simulink model "Open_Loop2024"  (R2025b)
settings: Solver=FixedStepAuto  StartTime=0.0  StopTime=10.0  FixedStep=0.0001  RelTol=1e-3  EnableMultiTasking=on
InitFcn:
  | Ts=100e-6;
  | 
  | Pair_poles=5;
  | 
  | PWM_frequesncy=10000;
  | 
  | Base_speed=4000;
  | 
  | motor.base_freq=100;
  | 
  | dataType = Simulink.NumericType;
  | 
  | dataType.DataTypeMode = 'Fixed-point: binary point scaling';
  | 
  | dataType.Signedness = 'Signed';
  | 
  | dataType.WordLength = 32;
  | 
  | dataType.FractionLength = 17;
undefined symbols (not defined in the file): DiscIntNeverNeededParam
libraries: stm32f4xxblockslib x14, stm32blockslib x2, mcbpositiondecoderlib x2, mcbcontrolslib x2, stm32f3xxblockslib x2
settings Model: STM32="{\"HardwareInterrupt\":[{\"ID\":\"Open_Loop2024:7\"},{\"ID\":\"Open_Loop2024:322\"}],\"DigitalPortWrite\":[{\"ID\":\"Open_Loop2024:136\"},{\"ID\":\"Open_Loop2024:394\"},{\"ID\":\"Open_Loop2024:286\"}],\"AnalogInput\":{\"ID\":\"Open_Loop2024:13\"},\"DigitalPortRead\":[{\"ID\":\"Open_Loop2024:219\"},{\"ID\":\"Open_Loop2024:220\"},{\"ID\":\"Open_Loop2024:221\"},{\"ID\":\"Open_Loop2024:342\"},{\"ID\":\"Open_Loop2024:343\"},{\"ID\":\"Open_Loop2024:344\"},{\"ID\":\"Open_Loop2024:366\"},{\"ID\":\"Open_Loop2024:367\"},{\"ID\":\"Open_Loop2024:368\"}],\"PWMOutput\":{\"ID\":\"Open_Loop2024:3\"},\"TimerCapture\":{\"ID\":\"Open_Loop2024:351\"},\"AnalogOutput\":{\"ID\":\"Open_Loop2024:377\"}}"  Creator=be125564  LastModifiedBy=be125564
settings SolverCC: AutoInsertRateTranBlk=on
settings OptimizationCC: DefaultParameterBehavior=Inlined  EnhancedBackFolding=on  PassReuseOutputArgsAs=Individual arguments  ZeroExternalMemoryAtStartup=off  ZeroInternalMemoryAtStartup=off  MaxStackSize=512  OptimizeBlockOrder=speed  DifferentSizesBufferReuse=on  OptimizationCustomize=off  EfficientTunableParamExpr=on
settings DebuggingCC: MultiTaskDSMMsg=warning  ParameterTunabilityLossMsg=error
settings HardwareCC: ProdBitPerPointer=32.0  ProdBitPerSizeT=32.0  ProdBitPerPtrDiffT=32.0  ProdLargestAtomicInteger=Long  ProdLargestAtomicFloat=Double  ProdWordSize=32.0  ProdLongLongMode=on  ProdHWDeviceType=ARM Compatible->ARM Cortex-M
settings SFSimCC: MATLABDynamicMemAlloc=off
settings RTWCC: SystemTargetFile=ert.tlc  HardwareBoard=STM32F3xx Based  TemplateMakefile=ert_default_tmf  Toolchain=GNU Tools for ARM Embedded Processors  Description=Embedded Coder
settings CodeAppCC: ForceParamTrailComments=on  IgnoreCustomStorageClasses=off  OperatorAnnotations=on  SimulinkDataObjDesc=on  SFDataObjDesc=on  InsertBlockDesc=on
settings ERTTargetCC: ExtModeTransport=3.0  ExtModeStaticAlloc=on  ExtModeStaticAllocSize=2048.0  ExtModeMexFile=ext_xcp  ExtModeIntrfLevel=Level2 - Open  DynamicArrayContainerType=coder::array  TargetLangStandard=C99 (ISO)  CodeReplacementLibrary=ARM Cortex-M

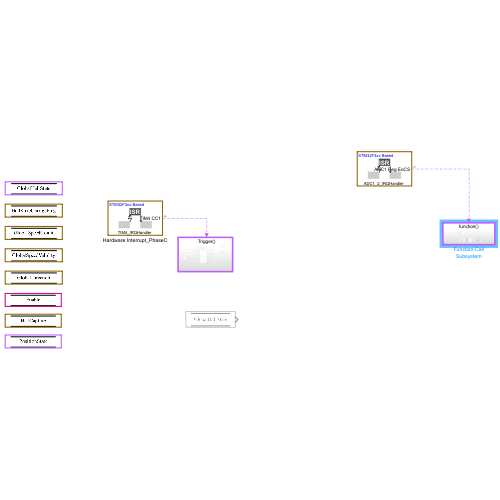
[thumbnail: Simulink's stored preview of the top-level diagram]
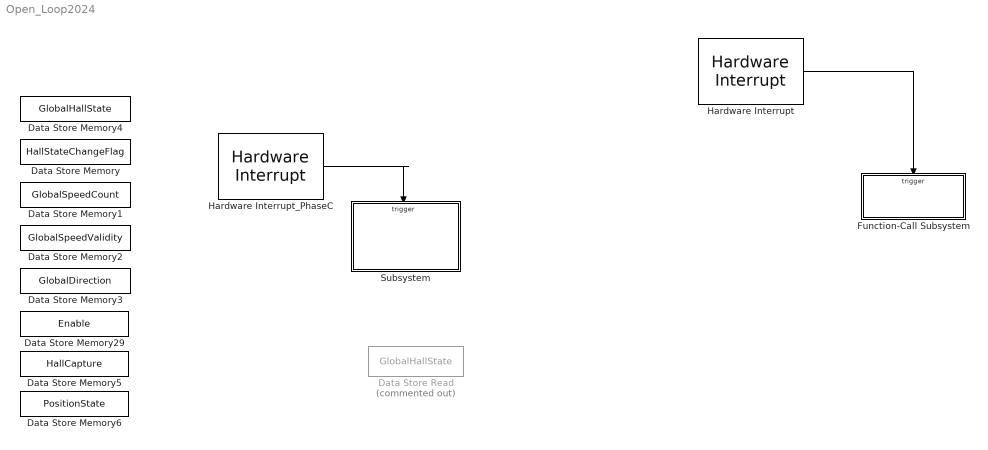
== system Open_Loop2024 ==
  Data Store Memory : DataStoreMemory  DataStoreName=HallStateChangeFlag  ShowAdditionalParam=off
  Data Store Memory1 : DataStoreMemory  DataStoreName=GlobalSpeedCount  ShowAdditionalParam=off
  Data Store Memory2 : DataStoreMemory  DataStoreName=GlobalSpeedValidity  ShowAdditionalParam=off
  Data Store Memory29 : DataStoreMemory  DataStoreName=Enable  ReadBeforeWriteMsg=warning  WriteAfterWriteMsg=warning  WriteAfterReadMsg=warning  ShowAdditionalParam=off  OutDataTypeStr=boolean
  Data Store Memory3 : DataStoreMemory  DataStoreName=GlobalDirection  ShowAdditionalParam=off
  Data Store Memory4 : DataStoreMemory  DataStoreName=GlobalHallState  ShowAdditionalParam=off  OutDataTypeStr=uint32
  Data Store Memory5 : DataStoreMemory  DataStoreName=HallCapture  ReadBeforeWriteMsg=warning  WriteAfterWriteMsg=warning  WriteAfterReadMsg=warning  ShowAdditionalParam=off  OutDataTypeStr=uint16
  Data Store Memory6 : DataStoreMemory  DataStoreName=PositionState  ReadBeforeWriteMsg=warning  WriteAfterWriteMsg=warning  WriteAfterReadMsg=warning  ShowAdditionalParam=off  OutDataTypeStr=uint16
  Data Store Read : DataStoreRead  Commented=on  DataStoreName=GlobalHallState  IndexOptions=Index vector (dialog)  Indices=1  OutputSizes=1
  Function-Call Subsystem : Subsystem  TreatAsAtomicUnit=on
  Hardware Interrupt : stm32f3xxblockslib/Hardware Interrupt  ISRGroup=Analog to digital converter (ADC)  ISRName=ADC1_2_IRQHandler  ISRNumber=33  EventsList={ 'off', 'ADC1 OVR', '1'; 'on', 'ADC1 Reg EoCS', '2'; 'off', 'ADC1 Watchdog1', '3'; 'off', 'ADC1 Watchdog2', '4'; 'off', 'ADC1 Watchdog3', '5'; 'off', 'ADC2 OVR', '6'; 'off', 'ADC2 Reg EoCS', '7'; 'off', 'ADC2 Watchdog1', '8'; 'off', 'ADC2 Watchdog2', '9'; 'off', 'ADC2 Watchdog3', '10'; 'off', 'Custom event', '11' }  SelectedEvents={'ADC1 Reg EoCS'}  TaskPriority=20  DisablePreemption=off  ClearInterruptFlagsAtEndOfEvent=on  InterruptDefinitionFile=$(TARGET_ROOT)/registry/interrupts/STM32F3xxBased_interrupts.xml  HardwareBoard=STM32F3xx Based  EnableSimPort=off
  Hardware Interrupt_PhaseC : stm32f3xxblockslib/Hardware Interrupt  ISRGroup=Timer (TIM)  ISRName=TIM4_IRQHandler  ISRNumber=45  EventsList={ 'off', 'TIM4 Update', '1'; 'on', 'TIM4 CC1', '2'; 'off', 'TIM4 CC2', '3'; 'off', 'TIM4 CC3', '4'; 'off', 'TIM4 CC4', '5'; 'off', 'TIM4 Trigger', '6'; 'off', 'Custom event', '7' }  SelectedEvents={'TIM4 CC1'}  TaskPriority=30  DisablePreemption=off  ClearInterruptFlagsAtEndOfEvent=on  InterruptDefinitionFile=$(TARGET_ROOT)/registry/interrupts/STM32F3xxBased_interrupts.xml  HardwareBoard=STM32F3xx Based  EnableSimPort=off
  Subsystem : Subsystem
  wires:
  Hardware Interrupt/1 -> Function-Call Subsystem/Trigger
  Hardware Interrupt_PhaseC/1 -> Subsystem/Trigger

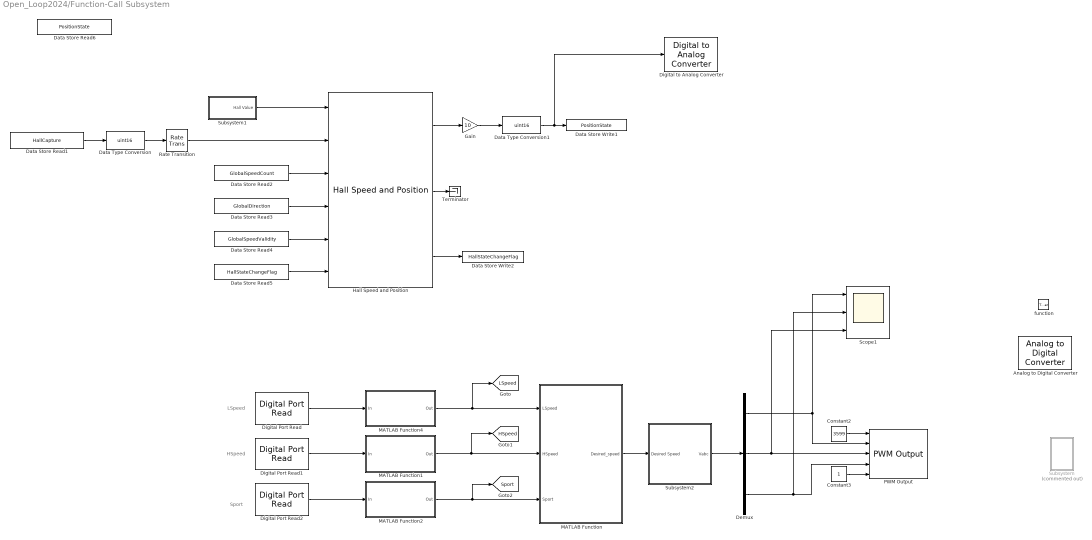
== system Open_Loop2024/Function-Call Subsystem ==
  note: Sport
  note: LSpeed
  note: HSpeed
  function : TriggerPort  TriggerType=function-call  VariantControl=(inherit)
  Analog to Digital Converter : stm32f4xxblockslib/Analog to Digital Converter  ADCModule=ADC1  ConversionGroup=Regular  TriggerMode=Trigger and read  NumberOfConversions=1  EnableBufferConv=off  BufferLength=1  OutputStatus=off  SampleTime=-1  EnableSimPort=off  hoistedMaskSrc=ECSoC/ECSimCodegen/Analog to Digital Converter
      settings: LibrarySourceBlock=stm32f3xxblockslib/Analog to Digital Converter
  Constant2 : Constant  Value=3599  SampleTime=-1
  Constant3 : Constant  SampleTime=-1
  Data Store Read1 : DataStoreRead  DataStoreName=HallCapture  IndexOptions=Index vector (dialog)  Indices=1  OutputSizes=1
  Data Store Read2 : DataStoreRead  DataStoreName=GlobalSpeedCount  IndexOptions=Index vector (dialog)  Indices=1  OutputSizes=1
  Data Store Read3 : DataStoreRead  DataStoreName=GlobalDirection  IndexOptions=Index vector (dialog)  Indices=1  OutputSizes=1
  Data Store Read4 : DataStoreRead  DataStoreName=GlobalSpeedValidity  IndexOptions=Index vector (dialog)  Indices=1  OutputSizes=1
  Data Store Read5 : DataStoreRead  Priority=1  DataStoreName=HallStateChangeFlag  IndexOptions=Index vector (dialog)  Indices=1  OutputSizes=1
  Data Store Read6 : DataStoreRead  DataStoreName=PositionState  IndexOptions=Index vector (dialog)  Indices=1  OutputSizes=1
  Data Store Write1 : DataStoreWrite  DataStoreName=PositionState  IndexOptions=Index vector (dialog)  Indices=1  OutputSizes=1
  Data Store Write2 : DataStoreWrite  DataStoreName=HallStateChangeFlag  IndexOptions=Index vector (dialog)  Indices=1  OutputSizes=1
  Data Type Conversion : DataTypeConversion  OutDataTypeStr=uint16  SaturateOnIntegerOverflow=off  RndMeth=Floor
  Data Type Conversion1 : DataTypeConversion  OutDataTypeStr=uint16  SaturateOnIntegerOverflow=off  RndMeth=Floor
  Demux : Demux  Outputs=3
  Digital Port Read : stm32f4xxblockslib/Digital Port Read  PortName=GPIOC  PinNumber=[6]  ReadOperation=on  IOAsArray=on  SampleTime=-1  EnableSimPort=off  hoistedMaskSrc=ECSoC/ECSimCodegen/Digital Port Read
  Digital Port Read1 : stm32f4xxblockslib/Digital Port Read  PortName=GPIOC  PinNumber=[9]  ReadOperation=on  IOAsArray=on  SampleTime=-1  EnableSimPort=off  hoistedMaskSrc=ECSoC/ECSimCodegen/Digital Port Read
  Digital Port Read2 : stm32f4xxblockslib/Digital Port Read  PortName=GPIOC  PinNumber=[15]  ReadOperation=on  IOAsArray=on  SampleTime=-1  EnableSimPort=off  hoistedMaskSrc=ECSoC/ECSimCodegen/Digital Port Read
  Digital to Analog Converter : stm32blockslib/Digital to Analog Converter  ExecutionOrder=Last  DACModule=DAC1  TriggerType=Write only  ChannelGroup=Channel2  waveGenEnable=off  waveType=Noise/Triangular  TriggerEnable=on  stepTriggerEnable=on  resetTriggerEnable=on  TrigConfig=Independent trigger  DataLength=12 bits  DataAlignment=Right alignment  dacEnable=off  OutputStatus=off
      settings: LibrarySourceBlock=stm32f3xxblockslib/Digital to Analog Converter
  Gain : Gain  Gain=10
  Hall Speed and Position : mcbpositiondecoderlib/Hall Speed and Position  blkExecutionType=Speed and position  CounterSize=16 bits  ClkFreq=1e6  BlkSampleTime=1e-4  PolePairs=5  MinSpeed=35  HallInterruptConfig=Every 60 Degrees  SpeedUnit=RPM  PerUnitSpeed=1000  SpeedDataType=single  hallSequence=ABC  Sequence=[5,4,6,2,3,1]  EnableSecondOrder=2nd Order  PositionUnit=Degrees  PositionDataType=single
      settings: LibrarySourceBlock=mcblib/Sensor Decoders/Hall Speed and Position
  MATLAB Function : MATLAB Function  TreatAsAtomicUnit=on
  MATLAB Function1 : MATLAB Function  TreatAsAtomicUnit=on
  MATLAB Function2 : MATLAB Function  TreatAsAtomicUnit=on
  MATLAB Function4 : MATLAB Function  TreatAsAtomicUnit=on
  PWM Output : stm32f4xxblockslib/PWM Output  ProcessorFamily=STM32F4  TimerModule=TIM1  DutycycleUnits=Counts  EnableChannel1=on  EnableCaptureCompare1Input=off  EnableCaptureCompare1ComplementaryInput=off  EnableOutputCompare1ModeInput=off  EnableChannel2=on  EnableCaptureCompare2Input=off  EnableCaptureCompare2ComplementaryInput=off  EnableOutputCompare2ModeInput=off  EnableChannel3=on  EnableCaptureCompare3Input=off  EnableCaptureCompare3ComplementaryInput=off  EnableOutputCompare3ModeInput=off  EnableChannel4=off  EnableCaptureCompare4Input=off  EnableCaptureCompare4ComplementaryInput=off  EnableOutputCompare4ModeInput=off  EnableChannel5=off  EnableCaptureCompare5Input=off  EnableOutputCompare5ModeInput=off  EnableChannel6=off  EnableCaptureCompare6Input=off  EnableOutputCompare6ModeInput=off  EnableCounterInput=off  EnableMainOutputInput=on  EnableFrequencyInput=on  SetRCAfterCE=off  OutputDirection=off  OutputMainOutputEnableStatus=off  SampleTime=0.1  EnableSimPort=off  EnableUpdateEvent=off  EnableCaptureCompare1Event=off  EnableCaptureCompare2Event=off  EnableCaptureCompare3Event=off  EnableCaptureCompare4Event=off  EnableTriggerEvent=off  EnableBreakEvent=off  EnableBreakEvent2=off  hoistedMaskSrc=ECSoC/ECSimCodegen/PWM Output
      settings: LibrarySourceBlock=stm32f3xxblockslib/PWM Output
  Rate Transition : RateTransition
  Scope1 : Scope  NumInputPorts=3
      settings: ActiveDisplayYMinimum=1528.94411  ActiveDisplayYMaximum=2070.05602  DataLoggingVariableName=ScopeData6
  Subsystem : Subsystem  Commented=on  TreatAsAtomicUnit=on
  Subsystem1 : Subsystem
  Subsystem2 : Subsystem
  Terminator : Terminator
  tag scope: HSpeed=global, LSpeed=global, Sport=global
  wires:
  Digital Port Read1/1 -> MATLAB Function1/1(In)
  MATLAB Function4/1(Out) -> [LSpeed], MATLAB Function/1(LSpeed)
  Constant2/1 -> PWM Output/1
  Demux/1 -> Scope1/1, PWM Output/2
  Demux/2 -> Scope1/3, PWM Output/3
  MATLAB Function2/1(Out) -> [Sport], MATLAB Function/3(Sport)
  Digital Port Read2/1 -> MATLAB Function2/1(In)
  Constant3/1 -> PWM Output/5
  Demux/3 -> Scope1/2, PWM Output/4
  MATLAB Function1/1(Out) -> [HSpeed], MATLAB Function/2(HSpeed)
  Subsystem2/1(Vabc) -> Demux/1
  Digital Port Read/1 -> MATLAB Function4/1(In)
  MATLAB Function/1(Desired_speed) -> Subsystem2/1(Desired Speed)
  Data Store Read4/1 -> Hall Speed and Position/5
  Data Store Read2/1 -> Hall Speed and Position/3
  Data Store Read5/1 -> Hall Speed and Position/6
  Data Store Read3/1 -> Hall Speed and Position/4
  Subsystem1/1(Hall Value) -> Hall Speed and Position/1
  Hall Speed and Position/3 -> Data Store Write2/1
  Data Store Read1/1 -> Data Type Conversion/1
  Hall Speed and Position/1 -> Gain/1
  Hall Speed and Position/2 -> Terminator/1
  Gain/1 -> Data Type Conversion1/1
  Data Type Conversion/1 -> Rate Transition/1
  Data Type Conversion1/1 -> Digital to Analog Converter/1, Data Store Write1/1
  Rate Transition/1 -> Hall Speed and Position/2

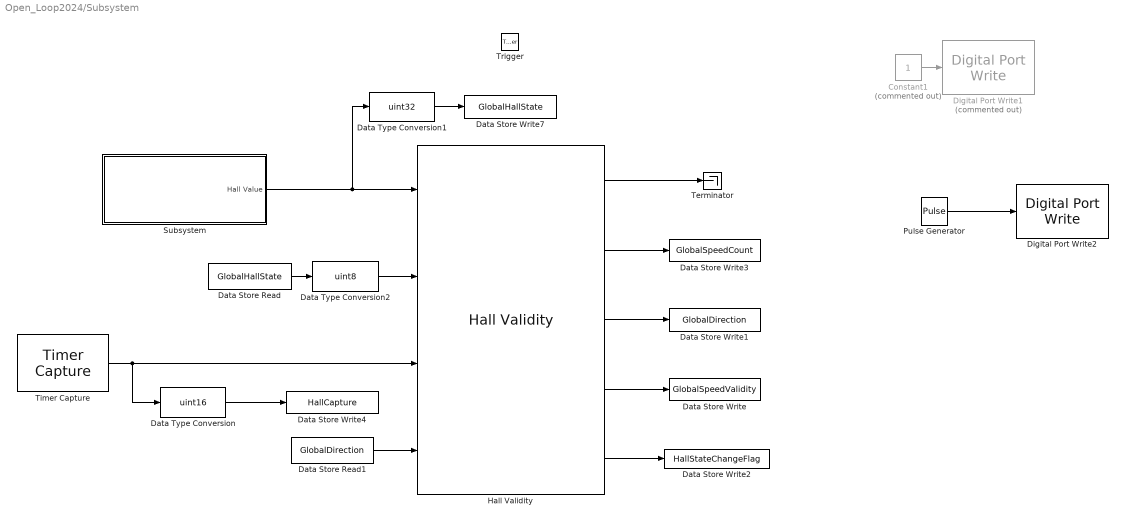
== system Open_Loop2024/Subsystem ==
  Trigger : TriggerPort  TriggerType=function-call  VariantControl=(inherit)  PortDimensions=1
  Constant1 : Constant  Commented=on  SampleTime=-1
  Data Store Read : DataStoreRead  DataStoreName=GlobalHallState  IndexOptions=Index vector (dialog)  Indices=1  OutputSizes=1
  Data Store Read1 : DataStoreRead  DataStoreName=GlobalDirection  IndexOptions=Index vector (dialog)  Indices=1  OutputSizes=1
  Data Store Write : DataStoreWrite  DataStoreName=GlobalSpeedValidity  IndexOptions=Index vector (dialog)  Indices=1  OutputSizes=1
  Data Store Write1 : DataStoreWrite  DataStoreName=GlobalDirection  IndexOptions=Index vector (dialog)  Indices=1  OutputSizes=1
  Data Store Write2 : DataStoreWrite  DataStoreName=HallStateChangeFlag  IndexOptions=Index vector (dialog)  Indices=1  OutputSizes=1
  Data Store Write3 : DataStoreWrite  DataStoreName=GlobalSpeedCount  IndexOptions=Index vector (dialog)  Indices=1  OutputSizes=1
  Data Store Write4 : DataStoreWrite  DataStoreName=HallCapture  IndexOptions=Index vector (dialog)  Indices=1  OutputSizes=1
  Data Store Write7 : DataStoreWrite  DataStoreName=GlobalHallState  IndexOptions=Index vector (dialog)  Indices=1  OutputSizes=1
  Data Type Conversion : DataTypeConversion  OutDataTypeStr=uint16  SaturateOnIntegerOverflow=off  RndMeth=Floor
  Data Type Conversion1 : DataTypeConversion  OutDataTypeStr=uint32  SaturateOnIntegerOverflow=off  RndMeth=Floor
  Data Type Conversion2 : DataTypeConversion  OutDataTypeStr=uint8  SaturateOnIntegerOverflow=off  RndMeth=Floor
  Digital Port Write1 : stm32f4xxblockslib/Digital Port Write  Commented=on  PortName=GPIOC  PinNumber=[11]  ReadOperation=off  IOAsArray=on  EnableSimPort=off  hoistedMaskSrc=ECSoC/ECSimCodegen/Digital Port Write
      settings: LibrarySourceBlock=stm32f3xxblockslib/Digital Port Write
  Digital Port Write2 : stm32f4xxblockslib/Digital Port Write  PortName=GPIOC  PinNumber=[11]  ReadOperation=off  IOAsArray=on  EnableSimPort=off  hoistedMaskSrc=ECSoC/ECSimCodegen/Digital Port Write
      settings: LibrarySourceBlock=stm32f3xxblockslib/Digital Port Write
  Hall Validity : mcbpositiondecoderlib/Hall Validity  hallSequence=ABC  sequence=[5,4,6,2,3,1]  CounterSize=16 bits
      settings: LibrarySourceBlock=mcblib/Sensor Decoders/Hall Validity
  Pulse Generator : DiscretePulseGenerator  SampleTime=-1
  Subsystem : Subsystem
  Terminator : Terminator
  Timer Capture : stm32blockslib/Timer Capture  TimerModule=TIM4  SelectedChannel=CH1  CaptureLength=1  OutputDataLength=off  OutputOverrunStatus=off  OutputDirection=off  SampleTime=-1
      settings: LibrarySourceBlock=stm32f3xxblockslib/Timer Capture
  wires:
  Subsystem/1(Hall Value) -> Data Type Conversion1/1, Hall Validity/1
  Timer Capture/1 -> Hall Validity/3, Data Type Conversion/1
  Data Store Read1/1 -> Hall Validity/4
  Hall Validity/5 -> Data Store Write2/1
  Hall Validity/1 -> Terminator/1
  Hall Validity/2 -> Data Store Write3/1
  Hall Validity/3 -> Data Store Write1/1
  Hall Validity/4 -> Data Store Write/1
  Data Store Read/1 -> Data Type Conversion2/1
  Data Type Conversion/1 -> Data Store Write4/1
  Data Type Conversion1/1 -> Data Store Write7/1
  Data Type Conversion2/1 -> Hall Validity/2
  Constant1/1 -> Digital Port Write1/1
  Pulse Generator/1 -> Digital Port Write2/1

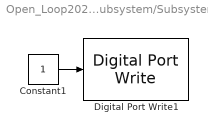
== system Open_Loop2024/Function-Call Subsystem/Subsystem ==
  Constant1 : Constant  SampleTime=-1
  Digital Port Write1 : stm32f4xxblockslib/Digital Port Write  PortName=GPIOC  PinNumber=[11]  ReadOperation=off  IOAsArray=on  EnableSimPort=off  hoistedMaskSrc=ECSoC/ECSimCodegen/Digital Port Write
      settings: LibrarySourceBlock=stm32f3xxblockslib/Digital Port Write
  wires:
  Constant1/1 -> Digital Port Write1/1

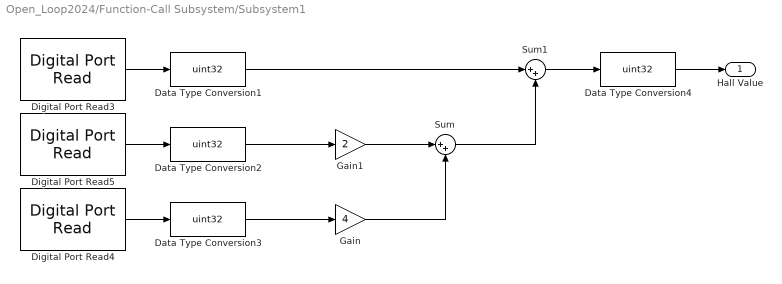
== system Open_Loop2024/Function-Call Subsystem/Subsystem1 ==
  Data Type Conversion{1..4} (4 alike) : DataTypeConversion  OutDataTypeStr=uint32  SaturateOnIntegerOverflow=off  RndMeth=Floor
  Digital Port Read3 : stm32f4xxblockslib/Digital Port Read  PortName=GPIOB  PinNumber=[8]  ReadOperation=on  IOAsArray=on  SampleTime=-1  EnableSimPort=off  hoistedMaskSrc=ECSoC/ECSimCodegen/Digital Port Read
  Digital Port Read4 : stm32f4xxblockslib/Digital Port Read  PortName=GPIOB  PinNumber=[7]  ReadOperation=on  IOAsArray=on  SampleTime=-1  EnableSimPort=off  hoistedMaskSrc=ECSoC/ECSimCodegen/Digital Port Read
  Digital Port Read5 : stm32f4xxblockslib/Digital Port Read  PortName=GPIOB  PinNumber=[6]  ReadOperation=on  IOAsArray=on  SampleTime=-1  EnableSimPort=off  hoistedMaskSrc=ECSoC/ECSimCodegen/Digital Port Read
  Gain : Gain  Gain=4
  Gain1 : Gain  Gain=2
  Sum : Sum  Inputs=|++
  Sum1 : Sum  Inputs=|++
  Hall Value : Outport
  wires:
  Digital Port Read4/1 -> Data Type Conversion3/1
  Gain1/1 -> Sum/1
  Sum/1 -> Sum1/2
  Gain/1 -> Sum/2
  Digital Port Read3/1 -> Data Type Conversion1/1
  Digital Port Read5/1 -> Data Type Conversion2/1
  Sum1/1 -> Data Type Conversion4/1
  Data Type Conversion1/1 -> Sum1/1
  Data Type Conversion3/1 -> Gain/1
  Data Type Conversion2/1 -> Gain1/1
  Data Type Conversion4/1 -> Hall Value/1

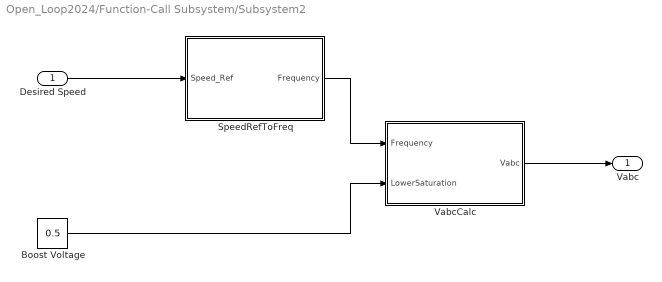
== system Open_Loop2024/Function-Call Subsystem/Subsystem2 ==
  Desired Speed : Inport
  Boost Voltage : Constant  Value=0.5  OutDataTypeStr=dataType  SampleTime=-1
  SpeedRefToFreq : Subsystem
  VabcCalc : Subsystem
  Vabc : Outport
  wires:
  Desired Speed/1 -> SpeedRefToFreq/1(Speed_Ref)
  SpeedRefToFreq/1(Frequency) -> VabcCalc/1(Frequency)
  Boost Voltage/1 -> VabcCalc/2(LowerSaturation)
  VabcCalc/1(Vabc) -> Vabc/1

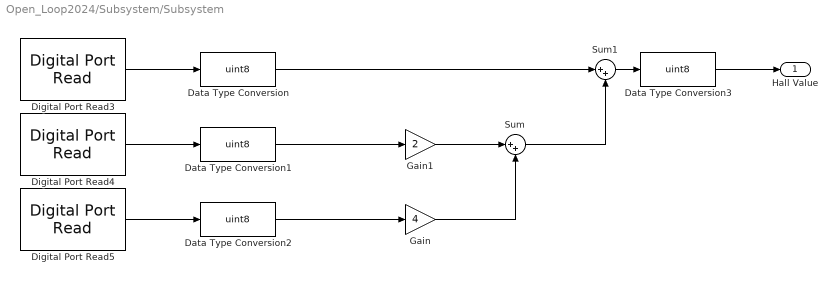
== system Open_Loop2024/Subsystem/Subsystem ==
  Data Type Conversion{,1..3} (4 alike) : DataTypeConversion  OutDataTypeStr=uint8  SaturateOnIntegerOverflow=off  RndMeth=Floor
  Digital Port Read3 : stm32f4xxblockslib/Digital Port Read  PortName=GPIOB  PinNumber=[8]  ReadOperation=on  IOAsArray=on  SampleTime=-1  EnableSimPort=off  hoistedMaskSrc=ECSoC/ECSimCodegen/Digital Port Read
      settings: LibrarySourceBlock=stm32f3xxblockslib/Digital Port Read
  Digital Port Read4 : stm32f4xxblockslib/Digital Port Read  PortName=GPIOB  PinNumber=[7]  ReadOperation=on  IOAsArray=on  SampleTime=-1  EnableSimPort=off  hoistedMaskSrc=ECSoC/ECSimCodegen/Digital Port Read
      settings: LibrarySourceBlock=stm32f3xxblockslib/Digital Port Read
  Digital Port Read5 : stm32f4xxblockslib/Digital Port Read  PortName=GPIOB  PinNumber=[6]  ReadOperation=on  IOAsArray=on  SampleTime=-1  EnableSimPort=off  hoistedMaskSrc=ECSoC/ECSimCodegen/Digital Port Read
      settings: LibrarySourceBlock=stm32f3xxblockslib/Digital Port Read
  Gain : Gain  Gain=4
  Gain1 : Gain  Gain=2
  Sum : Sum  Inputs=|++
  Sum1 : Sum  Inputs=|++
  Hall Value : Outport
  wires:
  Digital Port Read5/1 -> Data Type Conversion2/1
  Gain1/1 -> Sum/1
  Sum/1 -> Sum1/2
  Gain/1 -> Sum/2
  Digital Port Read3/1 -> Data Type Conversion/1
  Digital Port Read4/1 -> Data Type Conversion1/1
  Sum1/1 -> Data Type Conversion3/1
  Data Type Conversion/1 -> Sum1/1
  Data Type Conversion1/1 -> Gain1/1
  Data Type Conversion2/1 -> Gain/1
  Data Type Conversion3/1 -> Hall Value/1

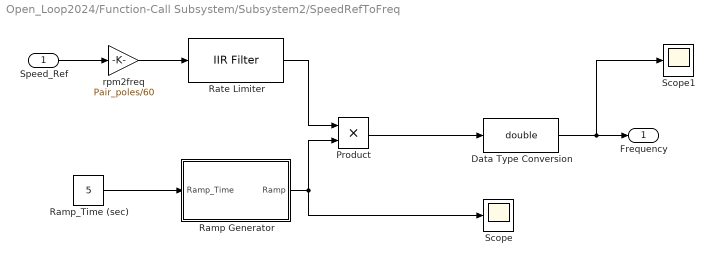
== system Open_Loop2024/Function-Call Subsystem/Subsystem2/SpeedRefToFreq ==
  Speed_Ref : Inport
  Data Type Conversion : DataTypeConversion  OutDataTypeStr=double  SaturateOnIntegerOverflow=off  RndMeth=Floor
  Product : Product  RndMeth=Simplest  OutDataTypeStr=Inherit: Same as first input
  Ramp Generator : Subsystem
  Ramp_Time (sec) : Constant  Value=5  OutDataTypeStr=dataType  SampleTime=-1
  Rate Limiter : mcbcontrolslib/IIR Filter  VariantControl=Low Pass Filter  VariantSelect=Low-pass  FilterConstantInputType=Specify via dialog  Filter_constant=0.0001  InitialOutput=Specify via dialog  InitialOutputValue=0  ExternalReset=none  advancedSettings=off  Ts=50e-6  cutOff_freq=0.31834
  Scope : Scope
      settings: ActiveDisplayYMinimum=-0.125  ActiveDisplayYMaximum=1.125  DataLoggingVariableName=ScopeData2
  Scope1 : Scope
      settings: ActiveDisplayYMinimum=-1.8558  ActiveDisplayYMaximum=16.7019  DataLoggingVariableName=ScopeData3
  rpm2freq : Gain  Gain=Pair_poles/60  OutDataTypeStr=dataType  RndMeth=Simplest
  Frequency : Outport
  wires:
  Data Type Conversion/1 -> Frequency/1, Scope1/1
  Rate Limiter/1 -> Product/1
  rpm2freq/1 -> Rate Limiter/1
  Ramp_Time (sec)/1 -> Ramp Generator/1(Ramp_Time)
  Ramp Generator/1(Ramp) -> Scope/1, Product/2
  Product/1 -> Data Type Conversion/1
  Speed_Ref/1 -> rpm2freq/1

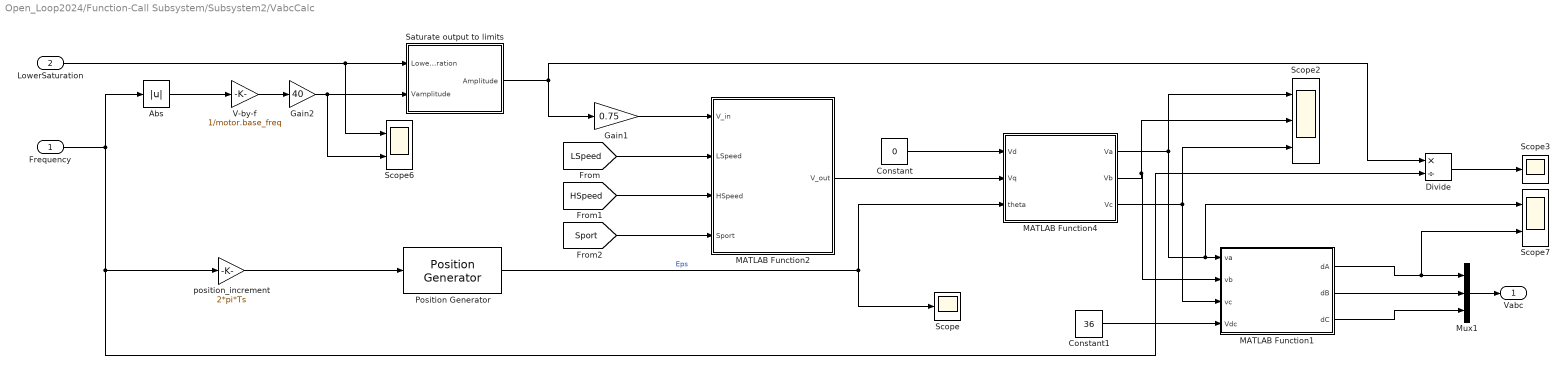
== system Open_Loop2024/Function-Call Subsystem/Subsystem2/VabcCalc ==
  Frequency : Inport
  LowerSaturation : Inport  Port=2
  Abs : Abs  RndMeth=Simplest  SaturateOnIntegerOverflow=off
  Constant : Constant  Value=0  SampleTime=-1
  Constant1 : Constant  Value=36  SampleTime=-1
  Divide : Product  Inputs=*/
  Gain1 : Gain  Gain=0.75
  Gain2 : Gain  Gain=40
  MATLAB Function1 : MATLAB Function  TreatAsAtomicUnit=on
  MATLAB Function2 : MATLAB Function  TreatAsAtomicUnit=on
  MATLAB Function4 : MATLAB Function  TreatAsAtomicUnit=on
  Mux1 : Mux  Inputs=3
  Position Generator : mcbcontrolslib/Position Generator  AngleOutput=Radians  InitialThetaSource=Specify via dialog  ExternalReset=none  Offset=0
  Saturate output to limits : Subsystem
  Scope : Scope
      settings: ActiveDisplayYMinimum=-0.2774  ActiveDisplayYMaximum=6.60459
  Scope2 : Scope  NumInputPorts=3
      settings: ActiveDisplayYMinimum=-3.125  ActiveDisplayYMaximum=3.125  DataLoggingVariableName=ScopeData2
  Scope3 : Scope
      settings: ActiveDisplayYMinimum=-4095.55  ActiveDisplayYMaximum=36863.95
  Scope6 : Scope  NumInputPorts=2
      settings: ActiveDisplayYMinimum=-0.54303  ActiveDisplayYMaximum=4.8873  DataLoggingVariableName=ScopeData4
  Scope7 : Scope  NumInputPorts=2
      settings: ActiveDisplayYMinimum=-3.066  ActiveDisplayYMaximum=3.047  DataLoggingVariableName=ScopeData5
  V-by-f : Gain  Gain=1/motor.base_freq  RndMeth=Simplest  OutDataTypeStr=Inherit: Same as input
  position_increment : Gain  Gain=2*pi*Ts  RndMeth=Simplest  OutDataTypeStr=Inherit: Same as input
  Vabc : Outport
  wires:
  Abs/1 -> V-by-f/1
  V-by-f/1 -> Gain2/1
  LowerSaturation/1 -> Scope6/1, Saturate output to limits/1(Lower Saturation)
  Mux1/1 -> Vabc/1
  position_increment/1 -> Position Generator/1
  MATLAB Function1/3(dC) -> Mux1/3
  MATLAB Function1/2(dB) -> Mux1/2
  MATLAB Function1/1(dA) -> Scope7/2, Mux1/1
  Frequency/1 -> Divide/2, position_increment/1, Abs/1
  Constant/1 -> MATLAB Function4/1(Vd)
  Position Generator/1 -> MATLAB Function4/3(theta), Scope/1  "Eps"
  MATLAB Function4/1(Va) -> Scope2/1, Scope7/1, MATLAB Function1/1(va)
  MATLAB Function4/2(Vb) -> MATLAB Function1/2(vb), Scope2/2
  MATLAB Function4/3(Vc) -> Scope2/3, MATLAB Function1/3(vc)
  Constant1/1 -> MATLAB Function1/4(Vdc)
  Divide/1 -> Scope3/1
  Saturate output to limits/1(Amplitude) -> Gain1/1, Divide/1
  Gain2/1 -> Scope6/2, Saturate output to limits/2(Vamplitude)
  [LSpeed] -> MATLAB Function2/2(LSpeed)
  [HSpeed] -> MATLAB Function2/3(HSpeed)
  [Sport] -> MATLAB Function2/4(Sport)
  Gain1/1 -> MATLAB Function2/1(V_in)
  MATLAB Function2/1(V_out) -> MATLAB Function4/2(Vq)

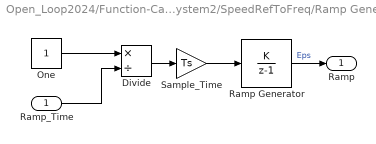
== system Open_Loop2024/Function-Call Subsystem/Subsystem2/SpeedRefToFreq/Ramp Generator ==
  Ramp_Time : Inport
  Divide : Product  Inputs=*/  RndMeth=Simplest  OutDataTypeStr=Inherit: Same as first input
  One : Constant  OutDataTypeStr=dataType  SampleTime=-1
  Ramp Generator : DiscreteIntegrator  IntegratorMethod=Accumulation: Forward Euler  gainval=1  SampleTime=-1  OutDataTypeStr=dataType  RndMeth=Simplest  LimitOutput=on  UpperSaturationLimit=1  LowerSaturationLimit=0  ICPrevOutput=DiscIntNeverNeededParam  ICPrevScaledInput=DiscIntNeverNeededParam
  Sample_Time : Gain  Gain=Ts  RndMeth=Simplest  OutDataTypeStr=Inherit: Same as input
  Ramp : Outport
  wires:
  Ramp_Time/1 -> Divide/2
  One/1 -> Divide/1
  Sample_Time/1 -> Ramp Generator/1
  Ramp Generator/1 -> Ramp/1  "Eps"
  Divide/1 -> Sample_Time/1

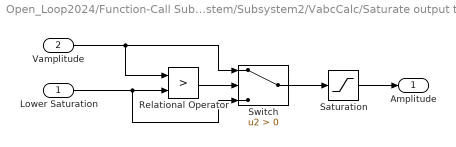
== system Open_Loop2024/Function-Call Subsystem/Subsystem2/VabcCalc/Saturate output to limits ==
  Lower Saturation : Inport
  Vamplitude : Inport  Port=2
  Relational Operator : RelationalOperator  Operator=>  OutDataTypeStr=boolean  RndMeth=Simplest  InputSameDT=off
  Saturation : Saturate  UpperLimit=20  LowerLimit=0  RndMeth=Simplest
  Switch : Switch  Criteria=u2 > Threshold  SaturateOnIntegerOverflow=off  InputSameDT=off
  Amplitude : Outport
  wires:
  Vamplitude/1 -> Relational Operator/1, Switch/1
  Relational Operator/1 -> Switch/2
  Switch/1 -> Saturation/1
  Saturation/1 -> Amplitude/1
  Lower Saturation/1 -> Relational Operator/2, Switch/3

== matlab function Open_Loop2024/Function-Call Subsystem/Subsystem2/VabcCalc/MATLAB Function4 ==
  data: Vd input; Va output; Vq input; theta input; Vb output; Vc output
function [Va, Vb, Vc] = dq_to_abc(Vd, Vq, theta)
%#codegen

% Normalize angle to [0, 2*pi] to be safe in codegen
theta = mod(single(theta), single(2*pi));

cos_t = cos(theta);
sin_t = sin(theta);

V_alpha = Vd * cos_t - Vq * sin_t;
V_beta  = Vd * sin_t + Vq * cos_t;

Va =  V_alpha;
Vb = -0.5 * V_alpha + 0.866 * V_beta;
Vc = -0.5 * V_alpha - 0.866 * V_beta;

== matlab function Open_Loop2024/Function-Call Subsystem/MATLAB Function ==
  data: LSpeed input; Desired_speed output; HSpeed input; Sport input
function Desired_speed = fcn(LSpeed, HSpeed, Sport)

Pair_poles=5;
if (LSpeed==1 && HSpeed==1 && Sport==1)
    val = (0*60)/Pair_poles;
   
elseif (LSpeed==1 && HSpeed==1 && Sport==0)
    val = (5*60)/Pair_poles;
  
elseif (LSpeed==1 && HSpeed==0 && Sport==0)
    val = (10*60)/Pair_poles;
   
elseif (LSpeed==0 && HSpeed==0 && Sport==0)
    val = (15*60)/Pair_poles;
     
elseif (LSpeed==0 && HSpeed==0 && Sport==1)
    val = (20*60)/Pair_poles;
elseif (LSpeed==0 && HSpeed==1 && Sport==1)
    val = (25*60)/Pair_poles;
elseif (LSpeed==0 && HSpeed==1 && Sport==0)
    val = (50*60)/Pair_poles;
else
    val = 0;
end

% Cast to sfix32_En17 (signed 32-bit, 17 fractional bits)
Desired_speed = fi(val, 1, 32, 17);

end

== matlab function Open_Loop2024/Function-Call Subsystem/MATLAB Function1 ==
  data: In input; Out output
function Out = debounce(In)
%#codegen
persistent stable_state
persistent counter

if isempty(stable_state)
    stable_state = In;
    counter = uint8(0);
end

DEBOUNCE_COUNT = uint8(5);  % adjust based on your sample rate

if In == stable_state
    counter = uint8(0);
else
    counter = counter + 1;
    if counter >= DEBOUNCE_COUNT
        stable_state = In;
        counter = uint8(0);
    end
end

Out = stable_state;
end

== matlab function Open_Loop2024/Function-Call Subsystem/Subsystem2/VabcCalc/MATLAB Function1 ==
  data: va input; dA output; vb input; vc input; Vdc input; dB output; dC output
function [dA,dB,dC] = svpwm(va, vb, vc, Vdc)
%#codegen
% Force single precision throughout
va  = single(va);
vb  = single(vb);
vc  = single(vc);
Vdc = single(Vdc);

% Constants (precise values, folded at compile time -> zero runtime cost)
TWO_THIRD = single(0.66666667);
SQRT3_2   = single(0.86602540);   % sqrt(3)/2
ARR       = single(3599);

% Clarke transform
Valpha = TWO_THIRD * (va - single(0.5)*vb - single(0.5)*vc);
Vbeta  = TWO_THIRD * (SQRT3_2*vb - SQRT3_2*vc);

% ---- Duty cycle times: direct (trig-free) method ----
% T1,T2 are exact linear combos of Valpha,Vbeta -> no atan2/sqrt/sin/floor.
invVdc = single(1) / Vdc;
C1 = single(1.5) * invVdc;   % 3/(2*Vdc)
C2 = SQRT3_2     * invVdc;   % sqrt(3)/(2*Vdc)

M1 = C1*Valpha - C2*Vbeta;
M2 = single(2)*C2*Vbeta;
M3 = M1 + M2;                % note: M3 = M1+M2 identically, only 3 valid sign patterns exist -> 6 sectors

sectorCode = uint8(M1>=single(0)) + uint8(2)*uint8(M2>=single(0)) + uint8(4)*uint8(M3>=single(0));

Ta = single(0); Tb = single(0); Tc = single(0);
switch sectorCode
    case uint8(7)   % sector 1
        T1=M1;  T2=M2;
        T0h=(single(1)-T1-T2)*single(0.5); T12=single(1)-T0h; T2h=T2+T0h; T1h=T1+T0h;
        Ta=T12; Tb=T2h; Tc=T0h;
    case uint8(6)   % sector 2
        T1=M3;  T2=-M1;
        T0h=(single(1)-T1-T2)*single(0.5); T12=single(1)-T0h; T2h=T2+T0h; T1h=T1+T0h;
        Ta=T1h; Tb=T12; Tc=T0h;
    case uint8(2)   % sector 3
        T1=M2;  T2=-M3;
        T0h=(single(1)-T1-T2)*single(0.5); T12=single(1)-T0h; T2h=T2+T0h; T1h=T1+T0h;
        Ta=T0h; Tb=T12; Tc=T2h;
    case uint8(0)   % sector 4
        T1=-M1; T2=-M2;
        T0h=(single(1)-T1-T2)*single(0.5); T12=single(1)-T0h; T2h=T2+T0h; T1h=T1+T0h;
        Ta=T0h; Tb=T1h; Tc=T12;
    case uint8(1)   % sector 5
        T1=-M3; T2=M1;
        T0h=(single(1)-T1-T2)*single(0.5); T12=single(1)-T0h; T2h=T2+T0h; T1h=T1+T0h;
        Ta=T2h; Tb=T0h; Tc=T12;
    otherwise       % sectorCode == 5, sector 6
        T1=-M2; T2=M3;
        T0h=(single(1)-T1-T2)*single(0.5); T12=single(1)-T0h; T2h=T2+T0h; T1h=T1+T0h;
        Ta=T12; Tb=T0h; Tc=T1h;
end

dA = ARR*Ta;
dB = ARR*Tb;
dC = ARR*Tc;
end

== matlab function Open_Loop2024/Function-Call Subsystem/MATLAB Function2 ==
  data: In input; Out output
function Out = debounce(In)
%#codegen
persistent stable_state
persistent counter

if isempty(stable_state)
    stable_state = In;
    counter = uint8(0);
end

DEBOUNCE_COUNT = uint8(5);  % adjust based on your sample rate

if In == stable_state
    counter = uint8(0);
else
    counter = counter + 1;
    if counter >= DEBOUNCE_COUNT
        stable_state = In;
        counter = uint8(0);
    end
end

Out = stable_state;
end

== matlab function Open_Loop2024/Function-Call Subsystem/Subsystem2/VabcCalc/MATLAB Function2 ==
  data: V_in input; V_out output; LSpeed input; HSpeed input; Sport input
function V_out = vf_saturation(V_in, LSpeed, HSpeed, Sport)
%#codegen
% Determines the saturation upper limit based on switch states
% (same switch logic as your speed-selection function), then
% saturates V_in between the fixed lower limit and that upper limit.

V_lower = 0.376; % fixed lower limit for all frequencies

if (LSpeed==1 && HSpeed==1 && Sport==1)
    V_upper = 0.376;   % 0 Hz -> standstill, output clamped to lower limit
elseif (LSpeed==1 && HSpeed==1 && Sport==0)
    V_upper = 1.2;     % 5 Hz
elseif (LSpeed==1 && HSpeed==0 && Sport==0)
    V_upper = 1.9;     % 10 Hz
elseif (LSpeed==0 && HSpeed==0 && Sport==0)
    V_upper = 2.5;     % 15 Hz
elseif (LSpeed==0 && HSpeed==0 && Sport==1)
    V_upper = 3.2;     % 20 Hz
elseif (LSpeed==0 && HSpeed==1 && Sport==1)
    V_upper = 4.0;     % 25 Hz
elseif (LSpeed==0 && HSpeed==1 && Sport==0)
    V_upper = 8.5;     % 50 Hz -- ESTIMATED, please replace with your real value
else
    V_upper = V_lower; % undefined switch combo -> safe fallback
end

% ---- Apply saturation ----
if V_in > V_upper
    V_out = V_upper;
elseif V_in < V_lower
    V_out = V_lower;
else
    V_out = V_in;
end

== matlab function Open_Loop2024/Function-Call Subsystem/MATLAB Function4 ==
  data: In input; Out output
function Out = debounce(In)
%#codegen
persistent stable_state
persistent counter

if isempty(stable_state)
    stable_state = In;
    counter = uint8(0);
end

DEBOUNCE_COUNT = uint8(5);  % adjust based on your sample rate

if In == stable_state
    counter = uint8(0);
else
    counter = counter + 1;
    if counter >= DEBOUNCE_COUNT
        stable_state = In;
        counter = uint8(0);
    end
end

Out = stable_state;
end
